simulink model "external_state_machine"  (R2021a)
settings: Solver=FixedStepDiscrete  StartTime=0.0  StopTime=2000*t_ADC  RelTol=1e-3
values from neighbouring files (symbols this model uses):
  A = 0.1    [uz_mpc_6ph_init.m]    (also in uz_mpc_6ph_state_machine_init.m)
  IB = sqrt(2)*IR    [uz_mpc_6ph_init.m]    (also in uz_mpc_6ph_state_machine_init.m)
  id_ref = 0.0    (= 0)    [uz_mpc_6ph_init.m]    (also in uz_mpc_6ph_state_machine_init.m)
  iq_ref = 15.0    (= 15)    [uz_mpc_6ph_init.m]    (also in uz_mpc_6ph_state_machine_init.m = 10)
  ix_ref = 0.0    (= 0)    [uz_mpc_6ph_init.m]    (also in uz_mpc_6ph_state_machine_init.m)
  iy_ref = 0.0    (= 0)    [uz_mpc_6ph_init.m]    (also in uz_mpc_6ph_state_machine_init.m)
  lambda_d = 1.0    (= 1)    [uz_mpc_6ph_init.m]    (also in uz_mpc_6ph_state_machine_init.m)
  lambda_q = 1.0    (= 1)    [uz_mpc_6ph_init.m]    (also in uz_mpc_6ph_state_machine_init.m)
  lambda_u = 0.0    (= 0)    [uz_mpc_6ph_init.m]    (also in uz_mpc_6ph_state_machine_init.m)
  lambda_x = 1.0    (= 1)    [uz_mpc_6ph_init.m]    (also in uz_mpc_6ph_state_machine_init.m)
  lambda_y = 1.0    (= 1)    [uz_mpc_6ph_init.m]    (also in uz_mpc_6ph_state_machine_init.m)
  Ld_over_LB = Ld/LB    [uz_mpc_6ph_init.m]    (also in uz_mpc_6ph_state_machine_init.m)
  Lq_over_LB = Lq/LB    [uz_mpc_6ph_init.m]    (also in uz_mpc_6ph_state_machine_init.m)
  n_rpm = 2200.0    (= 2200)    [uz_mpc_6ph_init.m]    (also in uz_mpc_6ph_state_machine_init.m = 100)
  omega_m = n_rpm*pi/30    (= 230.383461263)    [uz_mpc_6ph_init.m]    (also in uz_mpc_6ph_state_machine_init.m = 10.471975512)
  omegaB = nR*2*pi()/60*p    [uz_mpc_6ph_init.m]    (also in uz_mpc_6ph_state_machine_init.m)
  p = 5    [uz_mpc_6ph_init.m]    (also in uz_mpc_6ph_state_machine_init.m)
  psi_pm_over_psiB = psi_pm/psiB    [uz_mpc_6ph_init.m]    (also in uz_mpc_6ph_state_machine_init.m)
  Rs_over_ZB = Rs/ZB    [uz_mpc_6ph_init.m]    (also in uz_mpc_6ph_state_machine_init.m)
  t_ADC = 1/f_ADC    (= 1e-05)    [uz_mpc_6ph_init.m]    (also in uz_mpc_6ph_state_machine_init.m)
  t_clock = 1/f_clock    (= 1e-08)    [uz_mpc_6ph_init.m]    (also in uz_mpc_6ph_state_machine_init.m)
  Ts_times_ZB_over_Ld = Ts*ZB/Ld    [uz_mpc_6ph_init.m]    (also in uz_mpc_6ph_state_machine_init.m)
  Ts_times_ZB_over_Lq = Ts*ZB/Lq    [uz_mpc_6ph_init.m]    (also in uz_mpc_6ph_state_machine_init.m)
  Ts_times_ZB_over_Lx = Ts*ZB/Lx    [uz_mpc_6ph_init.m]    (also in uz_mpc_6ph_state_machine_init.m)
  Ts_times_ZB_over_Ly = Ts*ZB/Ly    [uz_mpc_6ph_init.m]    (also in uz_mpc_6ph_state_machine_init.m)
  v_dc = 565.0    (= 565)    [uz_mpc_6ph_init.m]    (also in uz_mpc_6ph_state_machine_init.m = 50)
  VB = sqrt(2/3)*VR    [uz_mpc_6ph_init.m]    (also in uz_mpc_6ph_state_machine_init.m)
libraries: nesl_utility x38, fl_lib x30, simulink x19, ee_lib x14, hdlsllib x4, spsAlphaBetaZerotodq0Lib x1
(part 2 of 4)

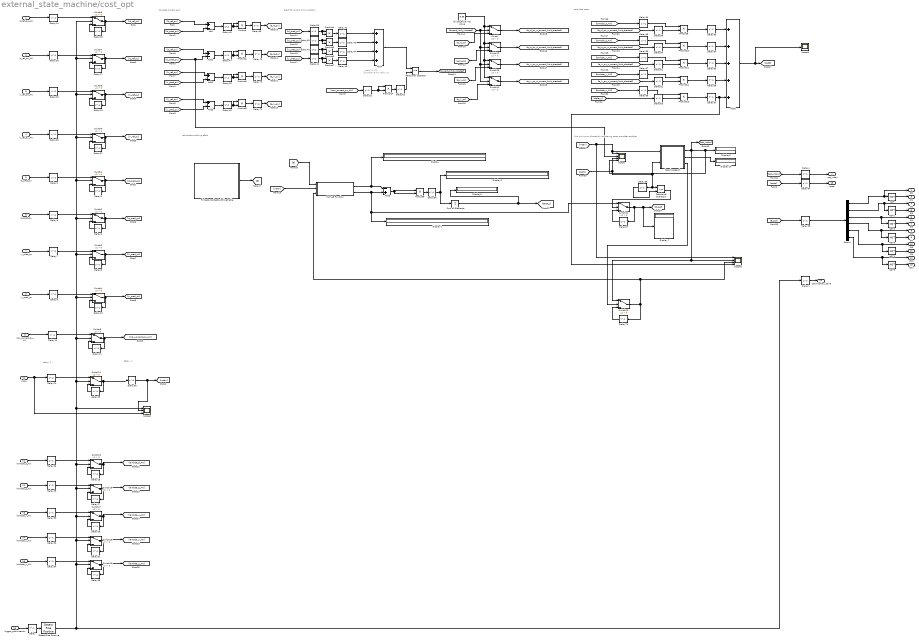
== system external_state_machine/cost_opt ==
  note: delay 4 !
  note: delay 2 !
  note: i_max^2 <= id^2+iq^2+ix^2+iy^2
  note: find minimum of costs by comparing costs one after another
  note: calculate costs
  note: calculate switching effort
  note: check for current limit violation
  note: squared current error
  id_ref_pu_AXI : Inport
  iq_ref_pu_AXI : Inport  Port=2
  ix_ref_pu_AXI : Inport  Port=3
  iy_ref_pu_AXI : Inport  Port=4
  id_pred_pu : Inport  Port=5
  iq_pred_pu : Inport  Port=6
  ix_pred_pu : Inport  Port=7
  iy_pred_pu : Inport  Port=8
  max_current_pu_AXI : Inport  Port=9
  index : Inport  Port=10
  lambda_d_AXI : Inport  Port=11
  lambda_q_AXI : Inport  Port=12
  lambda_x_AXI : Inport  Port=13
  lambda_y_AXI : Inport  Port=14
  lambda_u_AXI : Inport  Port=15
  trigger_optimization : Inport  Port=16
  Add{,1..3} (4 alike) : Sum  Inputs=+-
  Add4 : Sum  Inputs=++++  AccumDataTypeStr=fixdt_type_squared_current_error
  Add5 : Sum  Inputs=-+
  Add6 : Sum  Inputs=+++++  AccumDataTypeStr=fixdt_type_delta_u_costs
  Delay{,1..12,14..21,25..34,36,38..49,51..72,94} (67 alike) : Delay  DelayLength=1
  Delay23 : Delay  DelayLength=1  InitialCondition=1
  Delay24 : Delay  InitialCondition=1
  Delay35 : Delay  DelayLength=1  InitialCondition=4.99
  Delay37 : Delay  DelayLength=1  InitialCondition=0
  Delay50 : Delay  DelayLength=4  InitialCondition=1
  Delay73 : Delay  DelayLength=1  InitialCondition=1
  Demux : Demux  Outputs=6
  Detect Rise Positive : simulink/Logic and Bit Operations/Detect Rise Positive  vinit=0  OutDataTypeStr=boolean
  Display{,1..3,6..7,10} (7 alike) : Display
  FiniteControlSetSwitchingTable : MATLAB Function  TreatAsAtomicUnit=on
  MATLAB Function : MATLAB Function  TreatAsAtomicUnit=on
  NOT{,1..5} (6 alike) : Logic  Operator=NOT  IconShape=distinctive  AllPortsSameDT=off  OutDataTypeStr=boolean
  Product{,1..7,9..12,14} (13 alike) : Product  OutDataTypeStr=fixdt_type_squared_current_error
  Product13 : Product  OutDataTypeStr=fixdt_type_delta_u_costs
  Product8 : Product  OutDataTypeStr=uint16
  Relational Operator : RelationalOperator  OutDataTypeStr=boolean  RndMeth=Simplest
  Relational Operator1 : RelationalOperator  Operator=<=  OutDataTypeStr=boolean  RndMeth=Simplest
  Scope : Scope  NumInputPorts=4
  Scope1 : Scope  NumInputPorts=4
  Scope2 : Scope  NumInputPorts=3
  Scope3 : Scope
  Sum of Elements : Sum  Inputs=+  AccumDataTypeStr=uint16
  Switch{,1..9,11..21} (21 alike) : Switch  Criteria=u2 > Threshold
  iterativesearch : MATLAB Function  TreatAsAtomicUnit=on
  sfix18_En15 max value : Constant  Value=3.99  OutDataTypeStr=fixdt(1,18,15)  SampleTime=-1
  opt_index : Outport  VectorParamsAs1DForOutWhenUnconnected=off
  G0 : Outport  Port=2  VectorParamsAs1DForOutWhenUnconnected=off
  G1 : Outport  Port=3  VectorParamsAs1DForOutWhenUnconnected=off
  G2 : Outport  Port=4  VectorParamsAs1DForOutWhenUnconnected=off
  G3 : Outport  Port=5  VectorParamsAs1DForOutWhenUnconnected=off
  G4 : Outport  Port=6  VectorParamsAs1DForOutWhenUnconnected=off
  G5 : Outport  Port=7  VectorParamsAs1DForOutWhenUnconnected=off
  G6 : Outport  Port=8  VectorParamsAs1DForOutWhenUnconnected=off
  G7 : Outport  Port=9  VectorParamsAs1DForOutWhenUnconnected=off
  G8 : Outport  Port=10  VectorParamsAs1DForOutWhenUnconnected=off
  G9 : Outport  Port=11  VectorParamsAs1DForOutWhenUnconnected=off
  G10 : Outport  Port=12  VectorParamsAs1DForOutWhenUnconnected=off
  G11 : Outport  Port=13  VectorParamsAs1DForOutWhenUnconnected=off
  optimization_done : Outport  Port=14  VectorParamsAs1DForOutWhenUnconnected=off
  costs : Outport  Port=15  VectorParamsAs1DForOutWhenUnconnected=off
  wires:
  trigger_optimization/1 -> Delay/1
  Delay/1 -> Detect Rise Positive/1
  Delay1/1 -> optimization_done/1
  Delay4/1 -> opt_index/1
  Switch9/1 -> [iy_ref_pu], Delay21/1
  Delay17/1 -> Switch7/3
  id_ref_pu_AXI/1 -> Delay14/1
  Delay18/1 -> Switch8/1
  Switch8/1 -> [ix_ref_pu], Delay19/1
  Delay21/1 -> Switch9/3
  Switch7/1 -> [iq_ref_pu], Delay17/1
  iy_ref_pu_AXI/1 -> Delay20/1
  iq_ref_pu_AXI/1 -> Delay16/1
  Delay16/1 -> Switch7/1
  Delay19/1 -> Switch8/3
  Delay20/1 -> Switch9/1
  Delay15/1 -> Switch6/3
  Switch6/1 -> [id_ref_pu], Delay15/1
  ix_ref_pu_AXI/1 -> Delay18/1
  Delay14/1 -> Switch6/1
  Switch1/1 -> [id_pred_pu], Delay3/1
  ix_pred_pu/1 -> Delay7/1
  Delay9/1 -> Switch4/1
  Delay2/1 -> Switch1/1
  Delay8/1 -> Switch3/3
  Delay5/1 -> Switch2/1
  iy_pred_pu/1 -> Delay9/1
  iq_pred_pu/1 -> Delay5/1
  Switch3/1 -> Delay8/1, [ix_pred_pu]
  Delay10/1 -> Switch4/3
  Switch2/1 -> [iq_pred_pu], Delay6/1
  Delay7/1 -> Switch3/1
  Switch4/1 -> [iy_pred_pu], Delay10/1
  Delay6/1 -> Switch2/3
  Delay3/1 -> Switch1/3
  id_pred_pu/1 -> Delay2/1
  max_current_pu_AXI/1 -> Delay12/1
  Delay12/1 -> Switch5/1
  Delay11/1 -> Switch5/3
  Switch5/1 -> [max_current_pu_AXI], Delay11/1
  FiniteControlSetSwitchingTable/1(G) -> [G]
  Delay24/1 -> Switch11/1
  index/1 -> Scope2/3, Delay24/1
  Delay23/1 -> Switch11/3
  Switch11/1 -> Delay23/1, Delay50/1
  [e_id_pu] -> Switch/3
  [current_limit_violated] -> Switch13/2, Switch14/2, Switch12/2, Switch/2
  [e_iq_pu] -> Switch12/3
  [e_ix_pu] -> Switch13/3
  sfix18_En15 max value/1 -> Switch/1, Switch14/1, Switch13/1, Switch12/1
  [e_iy_pu] -> Switch14/3
  [G] -> MATLAB Function/1(in)
  Delay26/1 -> Switch15/1
  Delay25/1 -> Switch15/3
  Switch15/1 -> [lambda_d_AXI], Delay25/1
  lambda_d_AXI/1 -> Delay26/1
  lambda_q_AXI/1 -> Delay28/1
  Delay28/1 -> Switch16/1
  Switch16/1 -> [lambda_q_AXI], Delay27/1
  Delay27/1 -> Switch16/3
  lambda_y_AXI/1 -> Delay32/1
  Switch18/1 -> [lambda_y_AXI], Delay31/1
  Delay31/1 -> Switch18/3
  Delay32/1 -> Switch18/1
  lambda_x_AXI/1 -> Delay30/1
  Delay30/1 -> Switch17/1
  Switch17/1 -> [lambda_x_AXI], Delay29/1
  Delay29/1 -> Switch17/3
  Delay33/1 -> Switch19/3
  Switch19/1 -> [lambda_u_AXI], Delay33/1
  lambda_u_AXI/1 -> Delay34/1
  Delay34/1 -> Switch19/1
  [opt_index] -> Delay4/1
  Delay38/1 -> Demux/1
  Add4/1 -> Relational Operator/1
  NOT/1 -> G1/1
  Demux/1 -> G0/1, NOT/1
  NOT5/1 -> G11/1
  NOT4/1 -> G9/1
  NOT3/1 -> G7/1
  NOT2/1 -> G5/1
  NOT1/1 -> G3/1
  Demux/2 -> NOT1/1, G2/1
  Demux/3 -> NOT2/1, G4/1
  Demux/4 -> NOT3/1, G6/1
  Demux/5 -> NOT4/1, G8/1
  Demux/6 -> NOT5/1, G10/1
  Product8/1 -> Delay58/1
  Add5/1 -> Product8/1, Product8/2
  MATLAB Function/1(G_next) -> Display/1, Add5/1
  Product9/1 -> Delay53/1
  Product10/1 -> Delay54/1
  Product11/1 -> Delay55/1
  Product12/1 -> Delay56/1
  Product13/1 -> Delay57/1
  Add6/1 -> Scope3/1, [costs]
  [lambda_d_AXI] -> Delay64/1
  [lambda_q_AXI] -> Delay65/1
  [lambda_x_AXI] -> Delay66/1
  [lambda_y_AXI] -> Delay67/1
  [lambda_u_AXI] -> Delay68/1
  [delta_u] -> Delay63/1
  [e_id_pu_w_current_limit_checked] -> Delay59/1
  [e_iy_pu_w_current_limit_checked] -> Delay62/1
  [e_ix_pu_w_current_limit_checked] -> Delay61/1
  [e_iq_pu_w_current_limit_checked] -> Delay60/1
  [id_ref_pu] -> Add/1
  [id_pred_pu] -> Add/2
  [iq_pred_pu] -> Scope/2, Add1/2
  [iq_ref_pu] -> Add1/1
  [ix_ref_pu] -> Add2/1
  [ix_pred_pu] -> Add2/2
  [iy_ref_pu] -> Add3/1
  [iy_pred_pu] -> Add3/2
  Add3/1 -> Delay49/1
  Add1/1 -> Delay47/1
  Add2/1 -> Delay48/1
  Add/1 -> Delay46/1
  Product3/1 -> Delay72/1
  Product2/1 -> Delay71/1
  Product1/1 -> Delay70/1
  Product/1 -> Delay69/1
  Product4/1 -> Delay42/1
  Product5/1 -> Delay43/1
  Product6/1 -> Delay44/1
  Product7/1 -> Delay45/1
  [id_pred_pu] -> Delay36/1
  [iq_pred_pu] -> Delay39/1
  [ix_pred_pu] -> Delay40/1
  [iy_pred_pu] -> Delay41/1
  Relational Operator/1 -> [current_limit_violated]
  Switch14/1 -> [e_iy_pu_w_current_limit_checked]
  Switch13/1 -> [e_ix_pu_w_current_limit_checked]
  Switch12/1 -> [e_iq_pu_w_current_limit_checked]
  Switch/1 -> [e_id_pu_w_current_limit_checked]
  [max_current_pu_AXI] -> Delay51/1
  Product14/1 -> Delay52/1
  [costs] -> Delay94/1
  Delay94/1 -> costs/1
  Delay37/1 -> Switch21/3
  Switch21/1 -> Display7/1, [G_opt], Delay37/1
  Detect Rise Positive/1 -> Scope2/1, Switch4/2, Switch3/2, Switch2/2, Switch1/2, Switch6/2, Switch7/2, Switch8/2, Switch9/2, Switch5/2, Switch11/2, Switch15/2, Switch16/2, Switch17/2, Switch18/2, Switch19/2, Delay1/1
  [costs] -> Scope/3, Delay35/1, Relational Operator1/1, iterativesearch/2(cost)
  [index] -> Scope1/1, iterativesearch/1(index), Scope/1  "idx"
  Delay35/1 -> Relational Operator1/2
  Relational Operator1/1 -> Switch21/2
  [G_opt] -> Delay38/1
  Delay36/1 -> Product4/2, Product4/1
  Delay39/1 -> Product5/2, Product5/1
  Delay40/1 -> Product6/2, Product6/1
  Delay41/1 -> Product7/2, Product7/1
  Delay44/1 -> Add4/3
  Delay42/1 -> Add4/1
  Delay45/1 -> Add4/4
  Delay43/1 -> Add4/2
  Delay46/1 -> Product/1, Product/2
  Delay47/1 -> Product1/1, Product1/2
  Delay48/1 -> Product2/1, Product2/2
  Delay49/1 -> Product3/1, Product3/2
  Delay50/1 -> Scope2/2, [index]
  Delay51/1 -> Product14/1, Product14/2
  Delay52/1 -> Relational Operator/2
  Delay53/1 -> Add6/1
  Delay54/1 -> Add6/2
  Delay55/1 -> Add6/3
  Delay56/1 -> Add6/4
  Delay57/1 -> Add6/5, Scope1/4  "dU"
  Delay58/1 -> Sum of Elements/1, Display2/1
  Delay59/1 -> Product9/2
  Delay60/1 -> Product10/2
  Delay61/1 -> Product11/2
  Delay62/1 -> Product12/2
  Delay63/1 -> Product13/2
  Delay64/1 -> Product9/1
  Delay65/1 -> Product10/1
  Delay66/1 -> Product11/1
  Delay67/1 -> Product12/1
  Delay68/1 -> Product13/1
  Delay69/1 -> [e_id_pu]
  Delay70/1 -> [e_iq_pu]
  Delay71/1 -> [e_ix_pu]
  Delay72/1 -> [e_iy_pu]
  Sum of Elements/1 -> [delta_u], Display3/1
  Switch20/1 -> Delay73/1, MATLAB Function/3(last_optim_index), Scope1/3  "last_opt_idx"
  MATLAB Function/2(G_prev) -> Display1/1, Switch21/1, Add5/2
  Delay73/1 -> Switch20/3
  iterativesearch/1(opt_idx) -> Scope1/2, Switch20/1, Scope/4, Display6/1, [opt_index]  "opt_idx"
  iterativesearch/3(opt_done) -> Switch20/2
  iterativesearch/2(min_costs) -> Display10/1
  [index] -> MATLAB Function/2(index)

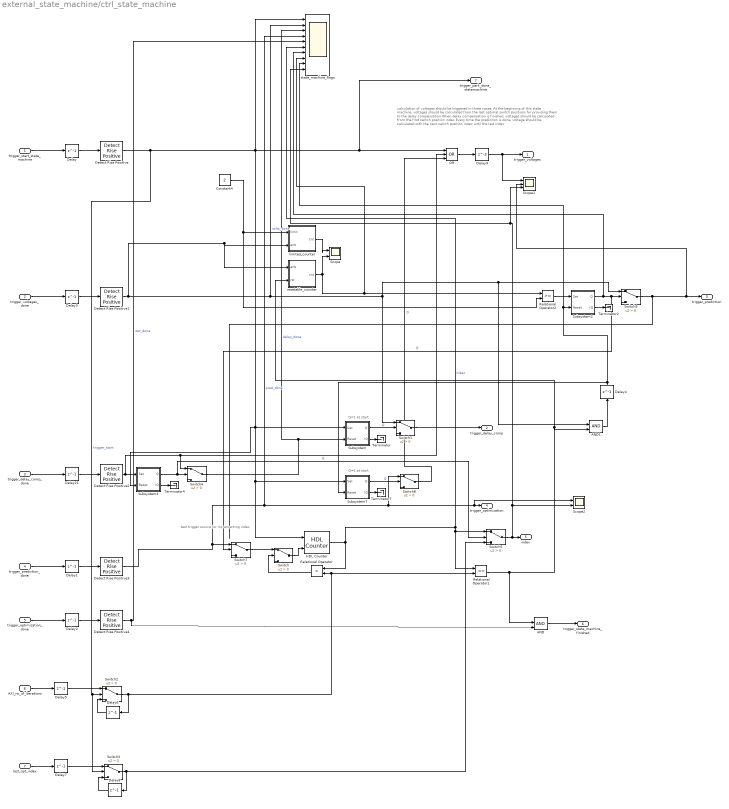
== system external_state_machine/ctrl_state_machine ==
  note: test trigger source for incrementing index
  note: calculation of voltages should be triggered in three cases:
      |
      | At the beginning of this state machine, voltages should be calculated from the last optimal switch positions for providing them to the delay compensation
      | When delay compensation is finished, voltages should be calculated from the first switch position index
      | Every time the prediciton is done, voltage should be calculated with the next switch position index until the last index
  note: Q=1 at start
  note: Q=1 at start
  trigger_start_state_machine : Inport
  trigger_voltages_done : Inport  Port=2
  trigger_delay_comp_done : Inport  Port=3
  trigger_prediction_done : Inport  Port=4
  trigger_optimization_done : Inport  Port=5
  AXI_no_of_iterations : Inport  Port=6  OutDataTypeStr=uint32
  last_opt_index : Inport  Port=7  OutDataTypeStr=uint32
  AND : Logic  IconShape=distinctive  AllPortsSameDT=off  OutDataTypeStr=boolean
  AND1 : Logic  IconShape=distinctive  AllPortsSameDT=off  OutDataTypeStr=boolean
  Constant4 : Constant  Value=2  OutDataTypeStr=uint8  SampleTime=-1
  Delay{,1..8,21} (10 alike) : Delay  DelayLength=1
  Delay9 : Delay  DelayLength=3
  Detect Rise Positive{,1..4} (5 alike) : simulink/Logic and Bit Operations/Detect Rise Positive  vinit=0  OutDataTypeStr=boolean
  HDL Counter : hdlsllib/Sources/HDL Counter  CountType=Free running  CountInit=1  CountStep=1  CountMax=25  CountFromType=Initial value  CountFrom=1  CountResetPort=on  CountLoadPort=off  CountEnbPort=on  CountDirPort=off  CountHitOutputPort=off  CountDataType=Unsigned  CountWordLen=32  CountFracLen=0  CountSampTime=1
  OR : Logic  Operator=OR  Inputs=3  IconShape=distinctive  AllPortsSameDT=off  OutDataTypeStr=boolean
  Relational Operator : RelationalOperator  Operator=<  OutDataTypeStr=boolean  RndMeth=Simplest
  Relational Operator1 : RelationalOperator  Operator===  OutDataTypeStr=boolean  RndMeth=Simplest
  Relational Operator2 : RelationalOperator  OutDataTypeStr=boolean  RndMeth=Simplest
  Scope : Scope  NumInputPorts=2
  Scope1 : Scope  NumInputPorts=3
  Scope2 : Scope  NumInputPorts=2
  Subsystem : Subsystem
  Subsystem2 : Subsystem
  Subsystem4 : Subsystem
  Subsystem7 : Subsystem
  Switch{,1..5,7..9} (9 alike) : Switch  Criteria=u2 > Threshold
  Terminator{,2,4,7} (4 alike) : Terminator
  limited_counter : Subsystem
  resetable_counter : Subsystem
  state_machine_flags : Scope  NumInputPorts=10
  trigger_voltages : Outport  VectorParamsAs1DForOutWhenUnconnected=off
  trigger_delay_comp : Outport  Port=2  VectorParamsAs1DForOutWhenUnconnected=off
  trigger_prediction : Outport  Port=3  VectorParamsAs1DForOutWhenUnconnected=off
  trigger_optimization : Outport  Port=4  VectorParamsAs1DForOutWhenUnconnected=off
  index : Outport  Port=5  VectorParamsAs1DForOutWhenUnconnected=off
  trigger_state_machine_finished : Outport  Port=6  VectorParamsAs1DForOutWhenUnconnected=off
  trigger_park_done_statemachine : Outport  Port=7  VectorParamsAs1DForOutWhenUnconnected=off
  wires:
  Switch2/1 -> Delay6/1, Relational Operator/2, Relational Operator1/2
  Relational Operator/1 -> Switch/2
  Detect Rise Positive/1 -> Switch3/2, Switch2/2, state_machine_flags/1, HDL Counter/1, Subsystem7/1(Set), Subsystem/1(Set), Subsystem4/2(Reset), trigger_park_done_statemachine/1, OR/1  "trigger_start"
  Subsystem/1(Q) -> Switch1/2  "Q"
  Subsystem/2(!Q) -> Terminator/1
  Switch1/1 -> trigger_delay_comp/1
  trigger_voltages_done/1 -> Delay3/1
  trigger_delay_comp_done/1 -> Delay21/1
  Delay21/1 -> Detect Rise Positive2/1
  Delay/1 -> Detect Rise Positive/1
  trigger_start_state_machine/1 -> Delay/1
  Delay2/1 -> Detect Rise Positive4/1
  trigger_optimization_done/1 -> Delay2/1
  Delay1/1 -> Detect Rise Positive3/1
  trigger_prediction_done/1 -> Delay1/1
  Subsystem4/1(Q) -> Switch5/2, Switch4/2  "Q"
  Subsystem4/2(!Q) -> Terminator4/1
  Detect Rise Positive2/1 -> OR/2, Switch4/1, Subsystem4/1(Set)
  Switch4/1 -> state_machine_flags/3, Subsystem/2(Reset)  "delay_done"
  Detect Rise Positive1/1 -> resetable_counter/1(enb), limited_counter/2(enb), state_machine_flags/2, AND1/1, Switch9/1, Switch1/1  "volts_done"
  Delay3/1 -> Detect Rise Positive1/1
  Subsystem2/2(!Q) -> Terminator2/1
  Subsystem2/1(Q) -> state_machine_flags/7, Switch7/2, Switch9/2  "Q"
  Constant4/1 -> Relational Operator2/2, limited_counter/1(limit)
  Relational Operator2/1 -> Subsystem2/1(Set)
  limited_counter/1(cnt) -> Scope/1
  Detect Rise Positive3/1 -> Switch7/1, state_machine_flags/4, Switch8/1, Scope2/1, trigger_optimization/1  "pred_done"
  Switch/1 -> HDL Counter/2
  HDL Counter/1 -> Switch5/1, Relational Operator1/1, state_machine_flags/6, Relational Operator/1  "index"
  Detect Rise Positive4/1 -> state_machine_flags/5, AND/2  "opt_done"
  Switch7/1 -> Switch/1
  resetable_counter/1(cnt) -> Scope/2, state_machine_flags/8, Relational Operator2/1
  Relational Operator1/1 -> AND1/2, resetable_counter/2(rst), AND/1
  Switch9/1 -> Scope1/2, trigger_prediction/1
  AND/1 -> trigger_state_machine_finished/1
  AND1/1 -> Delay4/1
  Delay4/1 -> state_machine_flags/9, Subsystem2/2(Reset), Subsystem7/2(Reset)
  Switch8/1 -> OR/3  "Q"
  Subsystem7/2(!Q) -> Terminator7/1
  Subsystem7/1(Q) -> Switch8/2  "Q"
  AXI_no_of_iterations/1 -> Delay5/1
  Delay5/1 -> Switch2/1
  Delay6/1 -> Switch2/3
  last_opt_index/1 -> Delay7/1
  Switch3/1 -> Switch5/3, Delay8/1
  Delay7/1 -> Switch3/1
  Delay8/1 -> Switch3/3
  Switch5/1 -> Scope1/3, state_machine_flags/10, Scope2/2, index/1
  OR/1 -> Delay9/1
  Delay9/1 -> Scope1/1, trigger_voltages/1

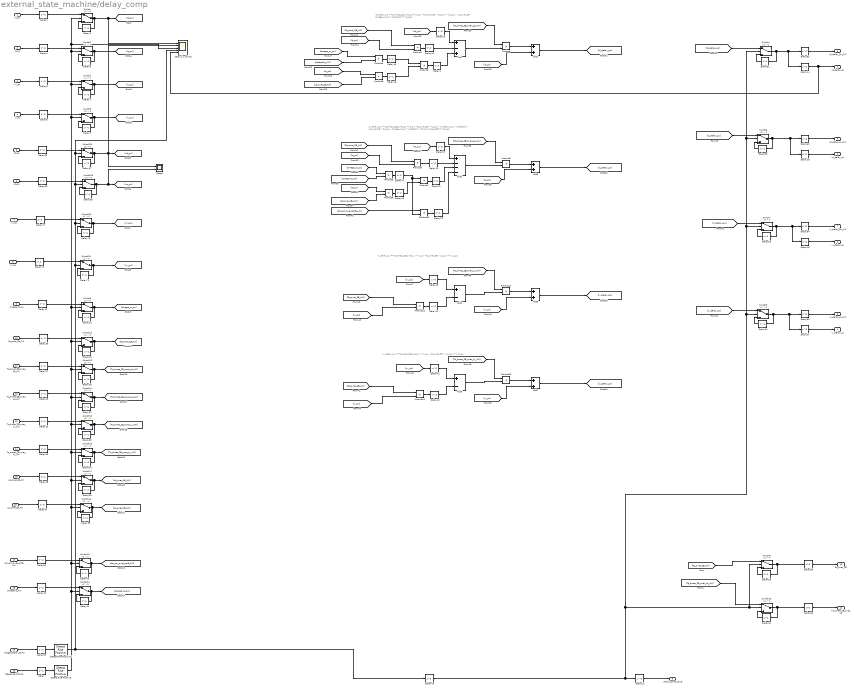
== system external_state_machine/delay_comp ==
  note: iy_delay_pu = Ts_times_ZB_over_Ly *(vy_pu - Rs_over_ZB * iy_k_pu) + iy_k_pu
  note: ix_delay_pu = Ts_times_ZB_over_Lx *(vx_pu - Rs_over_ZB* ix_k_pu) + ix_k_pu
  note: iq_delay_pu = Ts_times_ZB_over_Lq *(vq_pu - Rs_over_ZB * iq_k_pu - omega_m_pu * polepairs * Ld_over_LB * id_k_pu - omega_m_pu * polepairs * psi_pm_over_psiB) + iq_k_pu
  note: id_delay_pu = Ts_times_ZB_over_Ld *(vd_pu - Rs_over_ZB * id_k_pu + iq_k_pu * Lq_over_LB * omega_m_pu * polepairs) + id_k_pu
  id_pu : Inport  OutDataTypeStr=fixdt_type_dq_currents
  iq_pu : Inport  Port=2  OutDataTypeStr=fixdt_type_dq_currents
  ix_pu : Inport  Port=3  OutDataTypeStr=fixdt_type_xy_currents
  iy_pu : Inport  Port=4  OutDataTypeStr=fixdt_type_xy_currents
  vd_pu : Inport  Port=5  OutDataTypeStr=fixdt_type_dqxy_voltages
  vq_pu : Inport  Port=6  OutDataTypeStr=fixdt_type_dqxy_voltages
  vx_pu : Inport  Port=7  OutDataTypeStr=fixdt_type_dqxy_voltages
  vy_pu : Inport  Port=8  OutDataTypeStr=fixdt_type_dqxy_voltages
  omega_m_pu : Inport  Port=9  OutDataTypeStr=fixdt_type_speed
  Rs_over_ZB_AXI : Inport  Port=10  OutDataTypeStr=fixdt_type_constants
  Ts_times_ZB_over_Ld_AXI : Inport  Port=11  OutDataTypeStr=fixdt_type_constants
  Ts_times_ZB_over_Lq_AXI : Inport  Port=12  OutDataTypeStr=fixdt_type_constants
  Ts_times_ZB_over_Lx_AXI : Inport  Port=13  OutDataTypeStr=fixdt_type_constants
  Ts_times_ZB_over_Ly_AXI : Inport  Port=14  OutDataTypeStr=fixdt_type_constants
  Ld_over_LB_AXI : Inport  Port=15  OutDataTypeStr=fixdt_type_constants
  Lq_over_LB_AXI : Inport  Port=16  OutDataTypeStr=fixdt_type_constants
  psi_pm_over_psiB_AXI : Inport  Port=17  OutDataTypeStr=fixdt_type_constants
  polepairs_AXI : Inport  Port=18  OutDataTypeStr=fixdt_type_polepairs
  trigger_delay_comp : Inport  Port=19
  trigger_park_done : Inport  Port=20
  Add : Sum  Inputs=+-+  AccumDataTypeStr=fixdt(1,27,16)
  Add{1,3,5,7} (4 alike) : Sum  AccumDataTypeStr=fixdt(1,27,24)
  Add2 : Sum  Inputs=+---  AccumDataTypeStr=fixdt(1,27,16)
  Add4 : Sum  Inputs=+-  AccumDataTypeStr=fixdt(1,27,16)
  Add6 : Sum  Inputs=+-  AccumDataTypeStr=fixdt(1,27,16)
  Delay{,2,4,6,8,10..12,14..20,23..25,27,29,31,33,35,37,39,41..43,49..50,56,59..60,62..66,71,73} (40 alike) : Delay
  Delay{1,3,5,7,9,13,21..22,26,28,30,32,34,36,38,40,44..48,51..55,57..58,61,70,72} (31 alike) : Delay  DelayLength=1
  Detect Rise Positive : simulink/Logic and Bit Operations/Detect Rise Positive  vinit=0  OutDataTypeStr=boolean
  Detect Rise Positive1 : simulink/Logic and Bit Operations/Detect Rise Positive  vinit=0  OutDataTypeStr=boolean
  Product{,1..2,4..7,9..14} (13 alike) : Product  OutDataTypeStr=fixdt(1,18,15)
  Product3 : Product  OutDataTypeStr=fixdt(1,27,16)
  Product8 : Product  OutDataTypeStr=fixdt(1,27,16)
  Scope : Scope  NumInputPorts=2
  Switch : Switch  Criteria=u2 > Threshold  OutDataTypeStr=fixdt_type_dq_currents
  Switch1 : Switch  Criteria=u2 > Threshold  OutDataTypeStr=fixdt_type_dq_currents
  Switch{4,6..10} (6 alike) : Switch  Criteria=u2 > Threshold
  Switch{12..19} (8 alike) : Switch  Criteria=u2 > Threshold  OutDataTypeStr=fixdt_type_constants
  Switch2 : Switch  Criteria=u2 > Threshold  OutDataTypeStr=fixdt_type_xy_currents
  Switch21 : Switch  Criteria=u2 > Threshold  OutDataTypeStr=fixdt_type_polepairs
  Switch{28..31} (4 alike) : Switch  Criteria=u2 > Threshold  OutDataTypeStr=fixdt_type_dqxy_voltages
  Switch3 : Switch  Criteria=u2 > Threshold  OutDataTypeStr=fixdt_type_xy_currents
  Switch5 : Switch  Criteria=u2 > Threshold  OutDataTypeStr=fixdt_type_speed
  delay_in_values : Scope  NumInputPorts=5
  id_delay_pu : Outport
  iq_delay_pu : Outport  Port=2
  ix_delay_pu : Outport  Port=3
  iy_delay_pu : Outport  Port=4
  id_delay_pu_AXI : Outport  Port=5
  iq_delay_pu_AXI : Outport  Port=6
  ix_delay_pu_AXI : Outport  Port=7
  iy_delay_pu_AXI : Outport  Port=8
  delay_comp_done : Outport  Port=9
  Rs_over_ZB : Outport  Port=10
  Ts_times_ZB_over_Ld : Outport  Port=11
  wires:
  Add5/1 -> [ix_delay_pu]
  Switch12/1 -> [Rs_over_ZB_AXI], Delay26/1
  Add3/1 -> [iq_delay_pu]
  Add1/1 -> [id_delay_pu]
  Add7/1 -> [iy_delay_pu]
  Delay5/1 -> Switch1/3
  Delay25/1 -> Switch12/1
  Delay59/1 -> Switch28/1
  Delay33/1 -> Switch16/1
  vx_pu/1 -> Delay71/1
  vd_pu/1 -> Delay59/1
  Switch15/1 -> [Ts_times_ZB_over_Lx_AXI], Delay32/1
  Ld_over_LB_AXI/1 -> Delay35/1
  Delay2/1 -> Switch/1
  Switch16/1 -> Delay34/1, [Ts_times_ZB_over_Ly_AXI]
  ix_pu/1 -> Delay6/1
  Delay38/1 -> Switch18/3
  Switch17/1 -> Delay36/1, [Ld_over_LB_AXI]
  Delay9/1 -> Switch3/3
  Switch13/1 -> [Ts_times_ZB_over_Ld_AXI], Delay28/1
  Delay/1 -> Detect Rise Positive/1
  Delay34/1 -> Switch16/3
  Delay44/1 -> Switch21/3
  Delay29/1 -> Switch14/1
  Delay8/1 -> Switch3/1
  Switch29/1 -> Scope/2, [vq_pu], Delay58/1
  Switch3/1 -> [iy_pu], Delay9/1
  polepairs_AXI/1 -> Delay43/1
  Delay72/1 -> Switch31/3
  Delay43/1 -> Switch21/1
  Switch14/1 -> [Ts_times_ZB_over_Lq_AXI], Delay30/1
  Delay28/1 -> Switch13/3
  psi_pm_over_psiB_AXI/1 -> Delay39/1
  Delay58/1 -> Switch29/3
  id_pu/1 -> Delay2/1
  Switch21/1 -> [polepairs_AXI], Delay44/1
  Switch/1 -> delay_in_values/1, [id_pu], Delay3/1
  Delay35/1 -> Switch17/1
  Delay31/1 -> Switch15/1
  Switch28/1 -> Scope/1, delay_in_values/2, [vd_pu], Delay57/1
  Ts_times_ZB_over_Ly_AXI/1 -> Delay33/1
  Delay7/1 -> Switch2/3
  Delay37/1 -> Switch18/1
  Delay4/1 -> Switch1/1
  Switch2/1 -> [ix_pu], Delay7/1
  Delay12/1 -> Switch5/1
  Delay73/1 -> Switch31/1
  Switch31/1 -> Delay72/1, [vy_pu]
  omega_m_pu/1 -> Delay12/1
  Delay6/1 -> Switch2/1
  Delay27/1 -> Switch13/1
  vq_pu/1 -> Delay60/1
  Switch5/1 -> [omega_m_pu], Delay13/1
  Lq_over_LB_AXI/1 -> Delay37/1
  iq_pu/1 -> Delay4/1
  iy_pu/1 -> Delay8/1
  vy_pu/1 -> Delay73/1
  Delay70/1 -> Switch30/3
  Delay60/1 -> Switch29/1
  Switch30/1 -> Delay70/1, [vx_pu]
  Ts_times_ZB_over_Lq_AXI/1 -> Delay29/1
  Delay3/1 -> Switch/3
  Switch18/1 -> Delay38/1, [Lq_over_LB_AXI]
  Delay26/1 -> Switch12/3
  Switch19/1 -> [psi_pm_over_psiB_AXI], Delay40/1
  Ts_times_ZB_over_Lx_AXI/1 -> Delay31/1
  Delay71/1 -> Switch30/1
  Switch1/1 -> [iq_pu], Delay5/1
  Ts_times_ZB_over_Ld_AXI/1 -> Delay27/1
  Delay57/1 -> Switch28/3
  Rs_over_ZB_AXI/1 -> Delay25/1
  Delay39/1 -> Switch19/1
  trigger_park_done/1 -> Delay/1
  Delay40/1 -> Switch19/3
  Delay13/1 -> Switch5/3
  Delay32/1 -> Switch15/3
  Delay36/1 -> Switch17/3
  Delay30/1 -> Switch14/3
  Delay11/1 -> delay_comp_done/1
  Switch8/1 -> Delay54/1, Delay17/1, Delay65/1
  Switch4/1 -> Delay51/1, Delay14/1, Delay62/1
  Delay63/1 -> iq_delay_pu_AXI/1
  Delay65/1 -> iy_delay_pu_AXI/1
  Delay64/1 -> ix_delay_pu_AXI/1
  Switch7/1 -> Delay53/1, Delay16/1, Delay64/1
  Delay62/1 -> id_delay_pu_AXI/1
  Delay15/1 -> iq_delay_pu/1
  Delay14/1 -> delay_in_values/5, id_delay_pu/1
  Delay16/1 -> ix_delay_pu/1
  Delay17/1 -> iy_delay_pu/1
  Add/1 -> Product/2
  [Ts_times_ZB_over_Ld_AXI] -> Product/1  "Ts_times_ZB_over_Ld"
  Product/1 -> Add1/1
  [id_pu] -> Add1/2  "id_k_pu"
  [Rs_over_ZB_AXI] -> Product1/1  "Rs_over_ZB"
  [id_pu] -> Product1/2  "id_k_pu"
  [iq_pu] -> Product3/1  "iq_k_pu"
  [Lq_over_LB_AXI] -> Product3/2  "Lq_over_LB"
  [omega_m_pu] -> Product4/1  "omega_m_pu"
  [polepairs_AXI] -> Product4/2  "polepairs"
  [Ts_times_ZB_over_Lq_AXI] -> Product5/1  "Ts_times_ZB_over_Lq"
  [iq_pu] -> Product6/2  "iq_k_pu"
  [Rs_over_ZB_AXI] -> Product6/1  "Rs_over_ZB"
  Add2/1 -> Product5/2
  [omega_m_pu] -> Product9/1  "omega_m_pu"
  [iq_pu] -> Add3/2  "iq_k_pu"
  [id_pu] -> Product8/1  "id_k_pu"
  [Ld_over_LB_AXI] -> Product8/2  "Ld_over_LB"
  [polepairs_AXI] -> Product9/2  "polepairs"
  Product5/1 -> Add3/1
  [psi_pm_over_psiB_AXI] -> Product10/1
  [Ts_times_ZB_over_Lx_AXI] -> Product11/1  "Ts_times_ZB_over_Lx"
  [ix_pu] -> Product12/2  "ix_k_pu"
  [Rs_over_ZB_AXI] -> Product12/1  "Rs_over_ZB"
  Add4/1 -> Product11/2
  [ix_pu] -> Add5/2  "ix_k_pu"
  Product11/1 -> Add5/1
  [Rs_over_ZB_AXI] -> Product14/1  "Rs_over_ZB"
  Add6/1 -> Product13/2
  [iy_pu] -> Add7/2  "iy_k_pu"
  [iy_pu] -> Product14/2  "iy_k_pu"
  [Ts_times_ZB_over_Ly_AXI] -> Product13/1  "Ts_times_ZB_over_Ly"
  Product13/1 -> Add7/1
  Product2/1 -> Delay1/1
  Product1/1 -> Delay10/1
  Delay10/1 -> Add/2
  Delay1/1 -> Add/3
  [vd_pu] -> Delay18/1  "vd_pu"
  Delay18/1 -> Add/1
  [vq_pu] -> Delay19/1  "vq_pu"
  Product7/1 -> Delay21/1
  Product10/1 -> Delay22/1
  Delay22/1 -> Add2/4
  Delay21/1 -> Add2/3
  Delay20/1 -> Add2/2
  Delay19/1 -> Add2/1
  Product6/1 -> Delay20/1
  [vx_pu] -> Delay23/1  "vx_pu"
  Delay23/1 -> Add4/1
  Product12/1 -> Delay24/1
  Delay24/1 -> Add4/2
  [vy_pu] -> Delay41/1  "vy_pu"
  Product14/1 -> Delay42/1
  Delay42/1 -> Add6/2
  Delay41/1 -> Add6/1
  Product4/1 -> Delay45/1
  Product3/1 -> Delay46/1
  Delay46/1 -> Product2/2
  Delay45/1 -> Product2/1
  Product9/1 -> Delay47/1
  Delay47/1 -> Product10/2, Product7/1
  Product8/1 -> Delay48/1
  Delay48/1 -> Product7/2
  trigger_delay_comp/1 -> Delay50/1
  Delay50/1 -> Detect Rise Positive1/1
  Detect Rise Positive/1 -> Switch21/2, Switch19/2, Switch18/2, Switch17/2, Switch16/2, Switch15/2, Switch14/2, Switch13/2, Switch12/2, Switch5/2, Switch3/2, Switch2/2, Switch1/2, Switch/2, delay_in_values/3
  Detect Rise Positive1/1 -> Delay49/1, delay_in_values/4, Switch28/2, Switch29/2, Switch30/2, Switch31/2  "delay_comp done"
  [id_delay_pu] -> Switch4/1
  Delay51/1 -> Switch4/3
  [iq_delay_pu] -> Switch6/1
  Switch6/1 -> Delay52/1, Delay15/1, Delay63/1
  Delay52/1 -> Switch6/3
  [ix_delay_pu] -> Switch7/1
  Delay53/1 -> Switch7/3
  Delay54/1 -> Switch8/3
  [iy_delay_pu] -> Switch8/1
  Switch9/1 -> Delay55/1, Delay56/1
  Delay55/1 -> Switch9/3
  [Rs_over_ZB_AXI] -> Switch9/1
  Delay49/1 -> Switch9/2, Switch10/2, Switch8/2, Switch7/2, Switch6/2, Switch4/2, Delay11/1
  Delay56/1 -> Rs_over_ZB/1
  Switch10/1 -> Delay61/1, Delay66/1
  Delay61/1 -> Switch10/3
  [Ts_times_ZB_over_Ld_AXI] -> Switch10/1
  Delay66/1 -> Ts_times_ZB_over_Ld/1

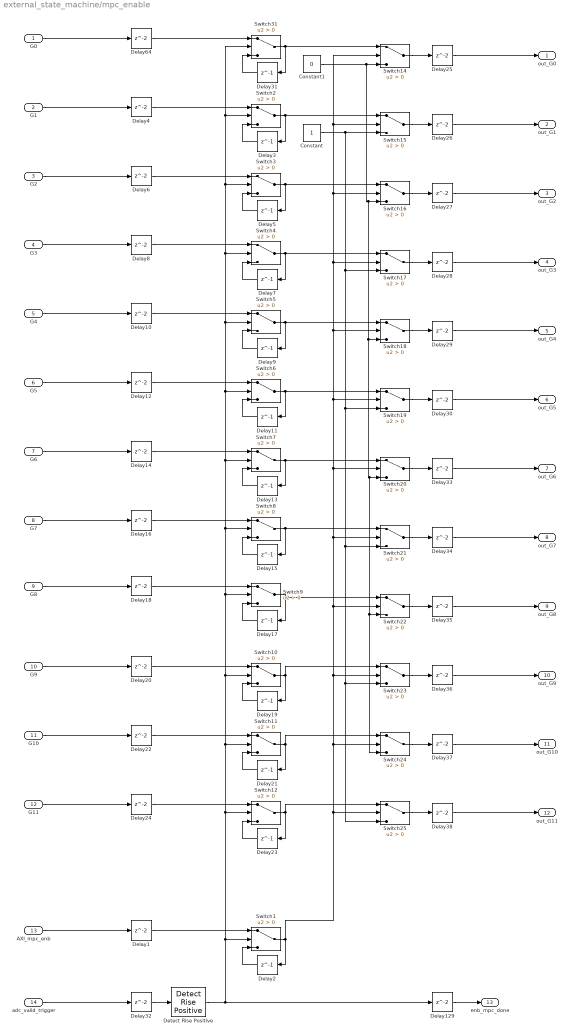
== system external_state_machine/mpc_enable ==
  G0 : Inport
  G1 : Inport  Port=2
  G2 : Inport  Port=3
  G3 : Inport  Port=4
  G4 : Inport  Port=5
  G5 : Inport  Port=6
  G6 : Inport  Port=7
  G7 : Inport  Port=8
  G8 : Inport  Port=9
  G9 : Inport  Port=10
  G10 : Inport  Port=11
  G11 : Inport  Port=12
  AXI_mpc_enb : Inport  Port=13
  adc_valid_trigger : Inport  Port=14  OutDataTypeStr=boolean
  Constant : Constant  OutDataTypeStr=boolean
  Constant1 : Constant  Value=0  OutDataTypeStr=boolean
  Delay{1,4,6,8,10,12,14,16,18,20,22,24..30,32..38,64,129} (27 alike) : Delay
  Delay{2..3,5,7,9,11,13,15,17,19,21,23,31} (13 alike) : Delay  DelayLength=1
  Detect Rise Positive : simulink/Logic and Bit Operations/Detect Rise Positive  vinit=0  OutDataTypeStr=boolean
  Switch{1..12,14..25,31} (25 alike) : Switch  Criteria=u2 > Threshold
  out_G0 : Outport
  out_G1 : Outport  Port=2
  out_G2 : Outport  Port=3
  out_G3 : Outport  Port=4
  out_G4 : Outport  Port=5
  out_G5 : Outport  Port=6
  out_G6 : Outport  Port=7
  out_G7 : Outport  Port=8
  out_G8 : Outport  Port=9
  out_G9 : Outport  Port=10
  out_G10 : Outport  Port=11
  out_G11 : Outport  Port=12
  enb_mpc_done : Outport  Port=13  OutDataTypeStr=boolean  LockScale=on
  wires:
  adc_valid_trigger/1 -> Delay32/1
  G0/1 -> Delay64/1
  Delay129/1 -> enb_mpc_done/1
  Delay64/1 -> Switch31/1
  Delay32/1 -> Detect Rise Positive/1
  Switch31/1 -> Switch14/1, Delay31/1
  Delay31/1 -> Switch31/3
  AXI_mpc_enb/1 -> Delay1/1
  Delay1/1 -> Switch1/1
  Delay2/1 -> Switch1/3
  Delay3/1 -> Switch2/3
  Switch2/1 -> Switch15/1, Delay3/1
  Delay4/1 -> Switch2/1
  G1/1 -> Delay4/1
  Detect Rise Positive/1 -> Delay129/1, Switch31/2, Switch2/2, Switch3/2, Switch4/2, Switch5/2, Switch6/2, Switch7/2, Switch8/2, Switch9/2, Switch10/2, Switch11/2, Switch12/2, Switch1/2
  Delay5/1 -> Switch3/3
  Switch3/1 -> Switch16/1, Delay5/1
  Delay6/1 -> Switch3/1
  G2/1 -> Delay6/1
  Delay7/1 -> Switch4/3
  Switch4/1 -> Switch17/1, Delay7/1
  Delay8/1 -> Switch4/1
  G3/1 -> Delay8/1
  Delay9/1 -> Switch5/3
  Switch5/1 -> Switch18/1, Delay9/1
  Delay10/1 -> Switch5/1
  G4/1 -> Delay10/1
  Delay11/1 -> Switch6/3
  Switch6/1 -> Switch19/1, Delay11/1
  Delay12/1 -> Switch6/1
  G5/1 -> Delay12/1
  Delay13/1 -> Switch7/3
  Switch7/1 -> Switch20/1, Delay13/1
  Delay14/1 -> Switch7/1
  G6/1 -> Delay14/1
  Delay15/1 -> Switch8/3
  Switch8/1 -> Switch21/1, Delay15/1
  Delay16/1 -> Switch8/1
  G7/1 -> Delay16/1
  Delay17/1 -> Switch9/3
  Switch9/1 -> Switch22/1, Delay17/1
  Delay18/1 -> Switch9/1
  G8/1 -> Delay18/1
  Delay19/1 -> Switch10/3
  Switch10/1 -> Delay19/1, Switch23/1
  Delay20/1 -> Switch10/1
  G9/1 -> Delay20/1
  Delay21/1 -> Switch11/3
  Switch11/1 -> Switch24/1, Delay21/1
  Delay22/1 -> Switch11/1
  G10/1 -> Delay22/1
  Delay23/1 -> Switch12/3
  Switch12/1 -> Switch25/1, Delay23/1
  Delay24/1 -> Switch12/1
  G11/1 -> Delay24/1
  Switch14/1 -> Delay25/1
  Delay25/1 -> out_G0/1
  Constant1/1 -> Switch24/3, Switch22/3, Switch20/3, Switch18/3, Switch16/3, Switch14/3
  Switch15/1 -> Delay26/1
  Delay26/1 -> out_G1/1
  Switch1/1 -> Switch25/2, Switch24/2, Switch23/2, Switch22/2, Switch21/2, Switch20/2, Switch19/2, Switch18/2, Switch17/2, Switch16/2, Switch15/2, Switch14/2, Delay2/1
  Switch16/1 -> Delay27/1
  Delay28/1 -> out_G3/1
  Switch17/1 -> Delay28/1
  Delay27/1 -> out_G2/1
  Delay29/1 -> out_G4/1
  Switch19/1 -> Delay30/1
  Switch18/1 -> Delay29/1
  Delay30/1 -> out_G5/1
  Switch22/1 -> Delay35/1
  Switch20/1 -> Delay33/1
  Delay35/1 -> out_G8/1
  Switch23/1 -> Delay36/1
  Delay33/1 -> out_G6/1
  Delay36/1 -> out_G9/1
  Delay38/1 -> out_G11/1
  Switch25/1 -> Delay38/1
  Switch24/1 -> Delay37/1
  Delay34/1 -> out_G7/1
  Delay37/1 -> out_G10/1
  Switch21/1 -> Delay34/1
  Constant/1 -> Switch25/3, Switch23/3, Switch21/3, Switch19/3, Switch17/3, Switch15/3

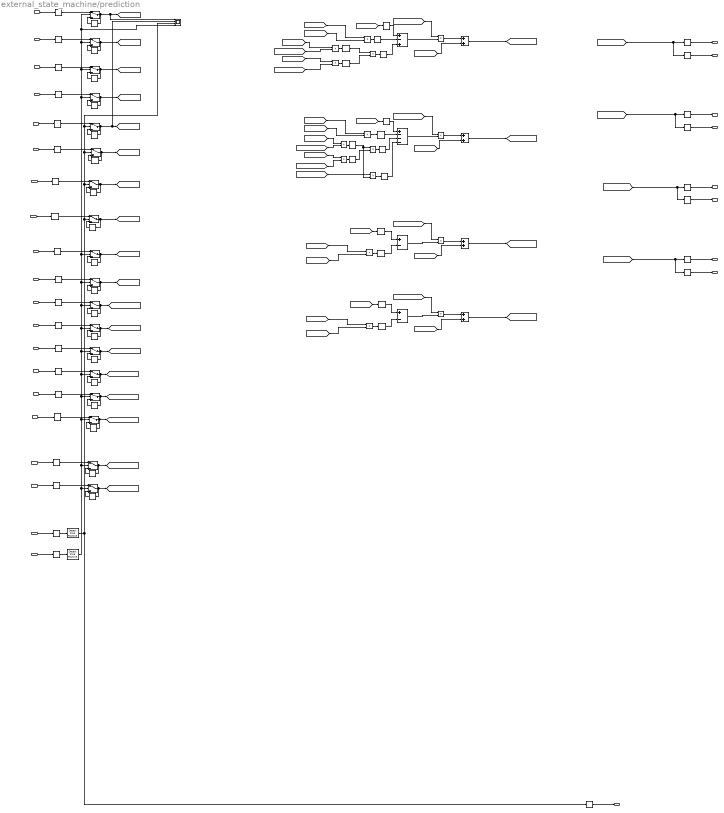
== system external_state_machine/prediction ==
  note: voltages are triggered every iteration
  note: iy_delay_pu = Ts_times_ZB_over_Ly *(vy_pu - Rs_over_ZB * iy_k_pu) + iy_k_pu
  note: ix_delay_pu = Ts_times_ZB_over_Lx *(vx_pu - Rs_over_ZB* ix_k_pu) + ix_k_pu
  note: iq_delay_pu = Ts_times_ZB_over_Lq *(vq_pu - Rs_over_ZB * iq_k_pu - omega_m_pu * polepairs * Ld_over_LB * id_k_pu - omega_m_pu * polepairs * psi_pm_over_psiB) + iq_k_pu
  note: id_delay_pu = Ts_times_ZB_over_Ld *(vd_pu - Rs_over_ZB * id_k_pu + iq_k_pu * Lq_over_LB * omega_m_pu * polepairs) + id_k_pu
  id_delay_pu : Inport  OutDataTypeStr=fixdt_type_dq_currents
  iq_delay_pu : Inport  Port=2  OutDataTypeStr=fixdt_type_dq_currents
  ix_delay_pu : Inport  Port=3  OutDataTypeStr=fixdt_type_dq_currents
  iy_delay_pu : Inport  Port=4  OutDataTypeStr=fixdt_type_dq_currents
  vd_pu : Inport  Port=5  OutDataTypeStr=fixdt_type_dqxy_voltages
  vq_pu : Inport  Port=6  OutDataTypeStr=fixdt_type_dqxy_voltages
  vx_pu : Inport  Port=7  OutDataTypeStr=fixdt_type_dqxy_voltages
  vy_pu : Inport  Port=8  OutDataTypeStr=fixdt_type_dqxy_voltages
  omega_m_pu : Inport  Port=9  OutDataTypeStr=fixdt_type_speed
  Rs_over_ZB_AXI : Inport  Port=10  OutDataTypeStr=fixdt_type_constants
  Ts_times_ZB_over_Ld_AXI : Inport  Port=11  OutDataTypeStr=fixdt_type_constants
  Ts_times_ZB_over_Lq_AXI : Inport  Port=12  OutDataTypeStr=fixdt_type_constants
  Ts_times_ZB_over_Lx_AXI : Inport  Port=13  OutDataTypeStr=fixdt_type_constants
  Ts_times_ZB_over_Ly_AXI : Inport  Port=14  OutDataTypeStr=fixdt_type_constants
  Ld_over_LB_AXI : Inport  Port=15  OutDataTypeStr=fixdt_type_constants
  Lq_over_LB_AXI : Inport  Port=16  OutDataTypeStr=fixdt_type_constants
  psi_pm_over_psiB_AXI : Inport  Port=17  OutDataTypeStr=fixdt_type_constants
  polepairs_AXI : Inport  Port=18  OutDataTypeStr=fixdt_type_polepairs
  trigger_prediction : Inport  Port=19
  trigger_delay_comp_done : Inport  Port=20
  Add : Sum  Inputs=+-+  AccumDataTypeStr=fixdt(1,27,16)
  Add{1,3,5,7} (4 alike) : Sum  AccumDataTypeStr=fixdt(1,27,24)
  Add2 : Sum  Inputs=+---  AccumDataTypeStr=fixdt(1,27,16)
  Add4 : Sum  Inputs=+-  AccumDataTypeStr=fixdt(1,27,16)
  Add6 : Sum  Inputs=+-  AccumDataTypeStr=fixdt(1,27,16)
  Delay{,2,4,6,8,11..12,14..17,25,27,29,31,33,35,37,39,43,50,59..60,62..65,71,73} (29 alike) : Delay
  Delay{1,3,5,7,9..10,13,18..24,26,28,30,32,34,36,38,40..42,44..48,57..58,70,72} (33 alike) : Delay  DelayLength=1
  Detect Rise Positive : simulink/Logic and Bit Operations/Detect Rise Positive  vinit=0  OutDataTypeStr=boolean
  Detect Rise Positive1 : simulink/Logic and Bit Operations/Detect Rise Positive  vinit=0  OutDataTypeStr=boolean
  Product{,1..2,4..7,9..14} (13 alike) : Product  OutDataTypeStr=fixdt(1,18,15)
  Product3 : Product  OutDataTypeStr=fixdt(1,27,16)
  Product8 : Product  OutDataTypeStr=fixdt(1,27,16)
  Scope : Scope  NumInputPorts=4
  Switch{,1..3} (4 alike) : Switch  Criteria=u2 > Threshold  OutDataTypeStr=fixdt_type_dq_currents
  Switch{12..19} (8 alike) : Switch  Criteria=u2 > Threshold  OutDataTypeStr=fixdt_type_constants
  Switch21 : Switch  Criteria=u2 > Threshold  OutDataTypeStr=fixdt_type_polepairs
  Switch{28..31} (4 alike) : Switch  Criteria=u2 > Threshold  OutDataTypeStr=fixdt_type_dqxy_voltages
  Switch5 : Switch  Criteria=u2 > Threshold  OutDataTypeStr=fixdt_type_speed
  id_pred_pu : Outport
  iq_pred_pu : Outport  Port=2
  ix_pred_pu : Outport  Port=3
  iy_pred_pu : Outport  Port=4
  id_pred_pu_AXI : Outport  Port=5
  iq_pred_pu_AXI : Outport  Port=6
  ix_pred_pu_AXI : Outport  Port=7
  iy_pred_pu_AXI : Outport  Port=8
  prediction_done : Outport  Port=9
  wires:
  Add5/1 -> [ix_delay_pu]
  Switch12/1 -> [Rs_over_ZB_AXI], Delay26/1
  Add3/1 -> [iq_delay_pu]
  Add1/1 -> [id_delay_pu]
  Add7/1 -> [iy_delay_pu]
  Delay5/1 -> Switch1/3
  Delay25/1 -> Switch12/1
  Delay59/1 -> Switch28/1
  Delay33/1 -> Switch16/1
  vx_pu/1 -> Delay71/1
  vd_pu/1 -> Delay59/1
  Switch15/1 -> [Ts_times_ZB_over_Lx_AXI], Delay32/1
  Ld_over_LB_AXI/1 -> Delay35/1
  Delay2/1 -> Switch/1
  Switch16/1 -> Delay34/1, [Ts_times_ZB_over_Ly_AXI]
  ix_delay_pu/1 -> Delay6/1
  Delay38/1 -> Switch18/3
  Switch17/1 -> Delay36/1, [Ld_over_LB_AXI]
  Delay9/1 -> Switch3/3
  Switch13/1 -> [Ts_times_ZB_over_Ld_AXI], Delay28/1
  Delay/1 -> Detect Rise Positive/1
  Delay34/1 -> Switch16/3
  Delay44/1 -> Switch21/3
  Delay29/1 -> Switch14/1
  Delay8/1 -> Switch3/1
  Switch29/1 -> [vq_pu], Delay58/1
  Switch3/1 -> [iy_pu], Delay9/1
  polepairs_AXI/1 -> Delay43/1
  Delay72/1 -> Switch31/3
  Delay43/1 -> Switch21/1
  Switch14/1 -> [Ts_times_ZB_over_Lq_AXI], Delay30/1
  Delay28/1 -> Switch13/3
  psi_pm_over_psiB_AXI/1 -> Delay39/1
  Delay58/1 -> Switch29/3
  id_delay_pu/1 -> Delay2/1
  Switch21/1 -> [polepairs_AXI], Delay44/1
  Switch/1 -> Scope/1, [id_pu], Delay3/1
  Delay35/1 -> Switch17/1
  Delay31/1 -> Switch15/1
  Switch28/1 -> Scope/2, [vd_pu], Delay57/1
  Ts_times_ZB_over_Ly_AXI/1 -> Delay33/1
  Delay7/1 -> Switch2/3
  Delay37/1 -> Switch18/1
  Delay4/1 -> Switch1/1
  Switch2/1 -> [ix_pu], Delay7/1
  Delay12/1 -> Switch5/1
  Delay73/1 -> Switch31/1
  Switch31/1 -> Delay72/1, [vy_pu]
  omega_m_pu/1 -> Delay12/1
  Delay6/1 -> Switch2/1
  Delay27/1 -> Switch13/1
  vq_pu/1 -> Delay60/1
  Switch5/1 -> [omega_m_pu], Delay13/1
  Lq_over_LB_AXI/1 -> Delay37/1
  iq_delay_pu/1 -> Delay4/1
  iy_delay_pu/1 -> Delay8/1
  vy_pu/1 -> Delay73/1
  Delay70/1 -> Switch30/3
  Delay60/1 -> Switch29/1
  Switch30/1 -> Delay70/1, [vx_pu]
  Ts_times_ZB_over_Lq_AXI/1 -> Delay29/1
  Delay3/1 -> Switch/3
  Switch18/1 -> Delay38/1, [Lq_over_LB_AXI]
  Delay26/1 -> Switch12/3
  Switch19/1 -> [psi_pm_over_psiB_AXI], Delay40/1
  Ts_times_ZB_over_Lx_AXI/1 -> Delay31/1
  Delay71/1 -> Switch30/1
  Switch1/1 -> [iq_pu], Delay5/1
  Ts_times_ZB_over_Ld_AXI/1 -> Delay27/1
  Delay57/1 -> Switch28/3
  Rs_over_ZB_AXI/1 -> Delay25/1
  Delay39/1 -> Switch19/1
  trigger_delay_comp_done/1 -> Delay/1
  Delay40/1 -> Switch19/3
  Delay13/1 -> Switch5/3
  Delay32/1 -> Switch15/3
  Delay36/1 -> Switch17/3
  Delay30/1 -> Switch14/3
  Delay11/1 -> prediction_done/1
  [iy_delay_pu] -> Delay17/1, Delay65/1
  [iq_delay_pu] -> Delay15/1, Delay63/1
  [id_delay_pu] -> Delay14/1, Delay62/1
  Delay63/1 -> iq_pred_pu_AXI/1
  Delay65/1 -> iy_pred_pu_AXI/1
  Delay64/1 -> ix_pred_pu_AXI/1
  [ix_delay_pu] -> Delay16/1, Delay64/1
  Delay62/1 -> id_pred_pu_AXI/1
  Delay15/1 -> iq_pred_pu/1
  Delay14/1 -> id_pred_pu/1
  Delay16/1 -> ix_pred_pu/1
  Delay17/1 -> iy_pred_pu/1
  Add/1 -> Product/2
  [Ts_times_ZB_over_Ld_AXI] -> Product/1  "Ts_times_ZB_over_Ld"
  Product/1 -> Add1/1
  [id_pu] -> Add1/2  "id_k_pu"
  [Rs_over_ZB_AXI] -> Product1/1  "Rs_over_ZB"
  [id_pu] -> Product1/2  "id_k_pu"
  [iq_pu] -> Product3/1  "iq_k_pu"
  [Lq_over_LB_AXI] -> Product3/2  "Lq_over_LB"
  [omega_m_pu] -> Product4/1  "omega_m_pu"
  [polepairs_AXI] -> Product4/2  "polepairs"
  [Ts_times_ZB_over_Lq_AXI] -> Product5/1  "Ts_times_ZB_over_Lq"
  [iq_pu] -> Product6/2  "iq_k_pu"
  [Rs_over_ZB_AXI] -> Product6/1  "Rs_over_ZB"
  Add2/1 -> Product5/2
  [omega_m_pu] -> Product9/1  "omega_m_pu"
  [iq_pu] -> Add3/2  "iq_k_pu"
  [id_pu] -> Product8/1  "id_k_pu"
  [Ld_over_LB_AXI] -> Product8/2  "Ld_over_LB"
  [polepairs_AXI] -> Product9/2  "polepairs"
  Product5/1 -> Add3/1
  [psi_pm_over_psiB_AXI] -> Product10/1
  [Ts_times_ZB_over_Lx_AXI] -> Product11/1  "Ts_times_ZB_over_Lx"
  [ix_pu] -> Product12/2  "ix_k_pu"
  [Rs_over_ZB_AXI] -> Product12/1  "Rs_over_ZB"
  Add4/1 -> Product11/2
  [ix_pu] -> Add5/2  "ix_k_pu"
  Product11/1 -> Add5/1
  [Rs_over_ZB_AXI] -> Product14/1  "Rs_over_ZB"
  Add6/1 -> Product13/2
  [iy_pu] -> Add7/2  "iy_k_pu"
  [iy_pu] -> Product14/2  "iy_k_pu"
  [Ts_times_ZB_over_Ly_AXI] -> Product13/1  "Ts_times_ZB_over_Ly"
  Product13/1 -> Add7/1
  Product2/1 -> Delay1/1
  Product1/1 -> Delay10/1
  Delay10/1 -> Add/2
  Delay1/1 -> Add/3
  [vd_pu] -> Delay18/1  "vd_pu"
  Delay18/1 -> Add/1
  [vq_pu] -> Delay19/1  "vq_pu"
  Product7/1 -> Delay21/1
  Product10/1 -> Delay22/1
  Delay22/1 -> Add2/4
  Delay21/1 -> Add2/3
  Delay20/1 -> Add2/2
  Delay19/1 -> Add2/1
  Product6/1 -> Delay20/1
  [vx_pu] -> Delay23/1  "vx_pu"
  Delay23/1 -> Add4/1
  Product12/1 -> Delay24/1
  Delay24/1 -> Add4/2
  [vy_pu] -> Delay41/1  "vy_pu"
  Product14/1 -> Delay42/1
  Delay42/1 -> Add6/2
  Delay41/1 -> Add6/1
  Product4/1 -> Delay45/1
  Product3/1 -> Delay46/1
  Delay46/1 -> Product2/2
  Delay45/1 -> Product2/1
  Product9/1 -> Delay47/1
  Delay47/1 -> Product10/2, Product7/1
  Product8/1 -> Delay48/1
  Delay48/1 -> Product7/2
  Detect Rise Positive1/1 -> Delay11/1, Switch31/2, Switch30/2, Switch29/2, Scope/3, Switch28/2  "delay_comp done"
  trigger_prediction/1 -> Delay50/1
  Delay50/1 -> Detect Rise Positive1/1
  Detect Rise Positive/1 -> Switch21/2, Switch19/2, Switch18/2, Switch17/2, Switch16/2, Switch15/2, Switch14/2, Switch13/2, Switch12/2, Switch5/2, Switch3/2, Switch2/2, Switch1/2, Scope/4, Switch/2

== system external_state_machine/pu_omega_m ==
  in1 : Inport  OutDataTypeStr=fixdt(1,24,11)
  AXI_pu_conv_in : Inport  Port=2  OutDataTypeStr=fixdt(0,18,18)
  adc_valid_trigger : Inport  Port=3  OutDataTypeStr=boolean
  Delay{32,64,127..129} (5 alike) : Delay
  Delay31 : Delay  DelayLength=1
  Detect Rise Positive : simulink/Logic and Bit Operations/Detect Rise Positive  vinit=0  OutDataTypeStr=boolean
  Product23 : Product  OutDataTypeStr=fixdt(1,24,11)
  Switch31 : Switch  Criteria=u2 > Threshold
  out1 : Outport
  pu_conv_done : Outport  Port=2  OutDataTypeStr=boolean  LockScale=on
  out1_AXI : Outport  Port=3
  wires:
  adc_valid_trigger/1 -> Delay32/1
  in1/1 -> Delay64/1
  Delay129/1 -> pu_conv_done/1
  AXI_pu_conv_in/1 -> Product23/1
  Delay64/1 -> Switch31/1
  Delay128/1 -> out1_AXI/1
  Delay32/1 -> Detect Rise Positive/1
  Switch31/1 -> Product23/2, Delay31/1
  Delay31/1 -> Switch31/3
  Detect Rise Positive/1 -> Delay129/1, Switch31/2
  Product23/1 -> Delay127/1, Delay128/1
  Delay127/1 -> out1/1

== system external_state_machine/pu_omega_m1 ==
  in1 : Inport  OutDataTypeStr=fixdt(1,24,11)
  AXI_pu_conv_in : Inport  Port=2  OutDataTypeStr=fixdt(0,18,18)
  adc_valid_trigger : Inport  Port=3  OutDataTypeStr=boolean
  Delay{32,64,127..129} (5 alike) : Delay
  Delay31 : Delay  DelayLength=1
  Detect Rise Positive : simulink/Logic and Bit Operations/Detect Rise Positive  vinit=0  OutDataTypeStr=boolean
  Product23 : Product  OutDataTypeStr=fixdt(1,24,11)
  Switch31 : Switch  Criteria=u2 > Threshold
  out1 : Outport
  pu_conv_done : Outport  Port=2  OutDataTypeStr=boolean  LockScale=on
  out1_AXI : Outport  Port=3
  wires:
  adc_valid_trigger/1 -> Delay32/1
  in1/1 -> Delay64/1
  Delay129/1 -> pu_conv_done/1
  AXI_pu_conv_in/1 -> Product23/1
  Delay64/1 -> Switch31/1
  Delay128/1 -> out1_AXI/1
  Delay32/1 -> Detect Rise Positive/1
  Switch31/1 -> Product23/2, Delay31/1
  Delay31/1 -> Switch31/3
  Detect Rise Positive/1 -> Delay129/1, Switch31/2
  Product23/1 -> Delay127/1, Delay128/1
  Delay127/1 -> out1/1

== system external_state_machine/pu_voltages_vsd ==
  note: 0=AXI 1=PL
  v_DC_pu : Inport  OutDataTypeStr=fixdt_type_constants
  sin_angle : Inport  Port=2  OutDataTypeStr=fixdt_type_sin_cos
  cos_angle : Inport  Port=3  OutDataTypeStr=fixdt_type_sin_cos
  index : Inport  Port=4
  index_select_AXI : Inport  Port=5
  index_AXI : Inport  Port=6
  trigger_park_done : Inport  Port=7
  trigger_voltages : Inport  Port=8
  Delay{,1,4..7,9..11,17..21} (14 alike) : Delay
  Delay12 : Delay  InitialCondition=1
  Delay13 : Delay  InitialCondition=1
  Delay14 : Delay  DelayLength=1  InitialCondition=1
  Delay15 : Delay  InitialCondition=1
  Delay16 : Delay  DelayLength=1  InitialCondition=1
  Delay2 : Delay  DelayLength=1
  Delay3 : Delay  DelayLength=1
  Delay56 : Delay  DelayLength=1
  Delay8 : Delay  DelayLength=1  InitialCondition=1
  Detect Rise Positive : simulink/Logic and Bit Operations/Detect Rise Positive  vinit=0  OutDataTypeStr=boolean
  Detect Rise Positive1 : simulink/Logic and Bit Operations/Detect Rise Positive  vinit=0  OutDataTypeStr=boolean
  Scope : Scope  NumInputPorts=2
  Switch : Switch  Criteria=u2 > Threshold
  Switch1 : Switch  Criteria=u2 > Threshold  OutDataTypeStr=fixdt_type_sin_cos
  Switch2 : Switch  Criteria=u2 > Threshold  OutDataTypeStr=fixdt_type_sin_cos
  Switch27 : Switch  Criteria=u2 > Threshold  OutDataTypeStr=fixdt_type_constants
  Switch3 : Switch  Criteria=u2 > Threshold  OutDataTypeStr=fixdt_type_polepairs
  Switch4 : Switch  Criteria=u2 > Threshold  OutDataTypeStr=fixdt_type_polepairs
  Switch5 : Switch  Criteria=u2 > Threshold  OutDataTypeStr=fixdt_type_polepairs
  finite_control_set : MATLAB Function  TreatAsAtomicUnit=on
  pu_vd : Outport
  pu_vq : Outport  Port=2
  pu_vx : Outport  Port=3
  pu_vy : Outport  Port=4
  pu_vd_AXI : Outport  Port=5
  pu_vq_AXI : Outport  Port=6
  pu_vx_AXI : Outport  Port=7
  pu_vy_AXI : Outport  Port=8
  voltages_done : Outport  Port=9
  wires:
  finite_control_set/1(pu_ud) -> Delay20/1, Delay7/1
  finite_control_set/2(pu_uq) -> Delay19/1, Delay6/1
  finite_control_set/3(pu_ux) -> Delay18/1, Delay5/1
  finite_control_set/4(pu_uy) -> Delay17/1, Delay4/1
  trigger_park_done/1 -> Delay/1
  Delay/1 -> Detect Rise Positive/1
  Delay56/1 -> Switch27/3
  v_DC_pu/1 -> Delay9/1
  Switch27/1 -> Delay56/1, finite_control_set/1(v_DC_pu)
  sin_angle/1 -> Delay10/1
  Delay2/1 -> Switch1/3
  Switch1/1 -> finite_control_set/2(sin_angle), Delay2/1
  cos_angle/1 -> Delay11/1
  Delay3/1 -> Switch2/3
  Switch2/1 -> finite_control_set/3(cos_angle), Delay3/1
  Delay4/1 -> pu_vy/1
  Delay5/1 -> pu_vx/1
  Delay6/1 -> pu_vq/1
  Delay7/1 -> pu_vd/1
  Switch3/1 -> Delay8/1, Switch/1
  index/1 -> Delay12/1
  Delay8/1 -> Switch3/3
  Delay9/1 -> Switch27/1
  Delay10/1 -> Switch1/1
  Delay11/1 -> Switch2/1
  Delay12/1 -> Switch3/1
  Delay14/1 -> Switch4/3
  index_AXI/1 -> Delay13/1
  Switch4/1 -> Switch/3, Delay14/1
  Delay13/1 -> Switch4/1
  Delay16/1 -> Switch5/3
  index_select_AXI/1 -> Delay15/1
  Switch5/1 -> Switch/2, Delay16/1
  Delay15/1 -> Switch5/1
  Delay17/1 -> pu_vy_AXI/1
  Delay19/1 -> pu_vq_AXI/1
  Delay20/1 -> pu_vd_AXI/1
  Delay18/1 -> pu_vx_AXI/1
  Detect Rise Positive1/1 -> Scope/2, Switch3/2, Switch4/2, Delay1/1  "trigger"
  Delay1/1 -> voltages_done/1
  Detect Rise Positive/1 -> Switch5/2, Switch2/2, Switch1/2, Switch27/2
  trigger_voltages/1 -> Delay21/1
  Delay21/1 -> Detect Rise Positive1/1
  Switch/1 -> Scope/1, finite_control_set/4(index)

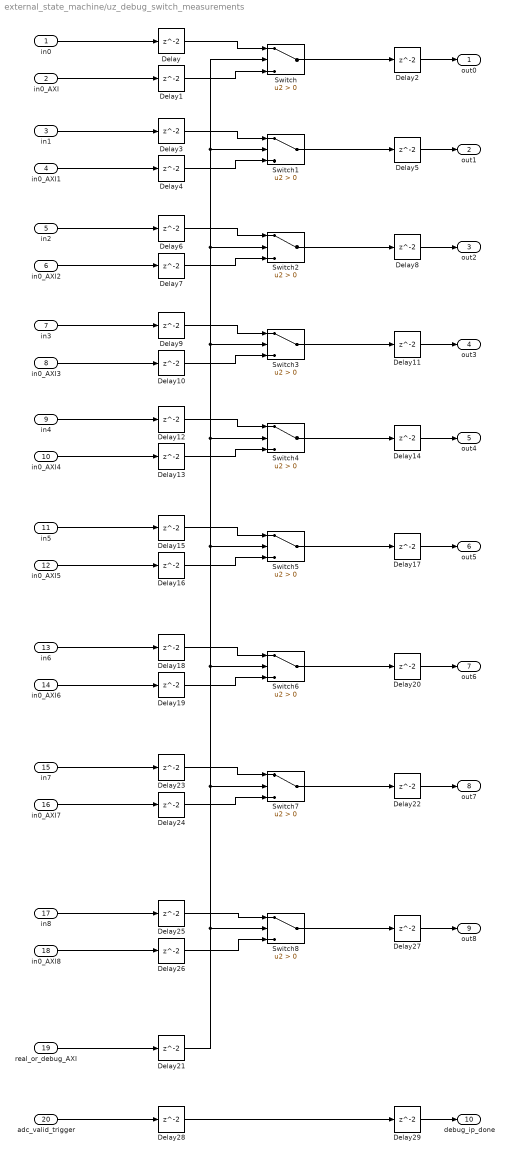
== system external_state_machine/uz_debug_switch_measurements ==
  in0 : Inport
  in0_AXI : Inport  Port=2
  in1 : Inport  Port=3
  in0_AXI1 : Inport  Port=4
  in2 : Inport  Port=5
  in0_AXI2 : Inport  Port=6
  in3 : Inport  Port=7
  in0_AXI3 : Inport  Port=8
  in4 : Inport  Port=9
  in0_AXI4 : Inport  Port=10
  in5 : Inport  Port=11
  in0_AXI5 : Inport  Port=12
  in6 : Inport  Port=13
  in0_AXI6 : Inport  Port=14
  in7 : Inport  Port=15
  in0_AXI7 : Inport  Port=16
  in8 : Inport  Port=17
  in0_AXI8 : Inport  Port=18
  real_or_debug_AXI : Inport  Port=19
  adc_valid_trigger : Inport  Port=20
  Delay{,1..29} (30 alike) : Delay
  Switch{,1..8} (9 alike) : Switch  Criteria=u2 > Threshold
  out0 : Outport  VectorParamsAs1DForOutWhenUnconnected=off
  out1 : Outport  Port=2  VectorParamsAs1DForOutWhenUnconnected=off
  out2 : Outport  Port=3  VectorParamsAs1DForOutWhenUnconnected=off
  out3 : Outport  Port=4  VectorParamsAs1DForOutWhenUnconnected=off
  out4 : Outport  Port=5  VectorParamsAs1DForOutWhenUnconnected=off
  out5 : Outport  Port=6  VectorParamsAs1DForOutWhenUnconnected=off
  out6 : Outport  Port=7  VectorParamsAs1DForOutWhenUnconnected=off
  out7 : Outport  Port=8  VectorParamsAs1DForOutWhenUnconnected=off
  out8 : Outport  Port=9  VectorParamsAs1DForOutWhenUnconnected=off
  debug_ip_done : Outport  Port=10  VectorParamsAs1DForOutWhenUnconnected=off
  wires:
  in0/1 -> Delay/1
  in0_AXI/1 -> Delay1/1
  Delay/1 -> Switch/1
  Delay1/1 -> Switch/3
  Switch/1 -> Delay2/1
  Delay2/1 -> out0/1
  in0_AXI1/1 -> Delay4/1
  Delay5/1 -> out1/1
  in1/1 -> Delay3/1
  Delay4/1 -> Switch1/3
  Delay3/1 -> Switch1/1
  Switch1/1 -> Delay5/1
  in0_AXI2/1 -> Delay7/1
  Delay8/1 -> out2/1
  in2/1 -> Delay6/1
  Delay7/1 -> Switch2/3
  Delay6/1 -> Switch2/1
  Switch2/1 -> Delay8/1
  in0_AXI3/1 -> Delay10/1
  Delay11/1 -> out3/1
  in3/1 -> Delay9/1
  Delay10/1 -> Switch3/3
  Delay9/1 -> Switch3/1
  Switch3/1 -> Delay11/1
  in0_AXI4/1 -> Delay13/1
  Delay14/1 -> out4/1
  in4/1 -> Delay12/1
  Delay13/1 -> Switch4/3
  Delay12/1 -> Switch4/1
  Switch4/1 -> Delay14/1
  in0_AXI5/1 -> Delay16/1
  Delay17/1 -> out5/1
  in5/1 -> Delay15/1
  Delay16/1 -> Switch5/3
  Delay15/1 -> Switch5/1
  Switch5/1 -> Delay17/1
  in0_AXI6/1 -> Delay19/1
  Delay20/1 -> out6/1
  in6/1 -> Delay18/1
  Delay19/1 -> Switch6/3
  Delay18/1 -> Switch6/1
  Switch6/1 -> Delay20/1
  real_or_debug_AXI/1 -> Delay21/1
  Delay22/1 -> out7/1
  Delay23/1 -> Switch7/1
  Delay24/1 -> Switch7/3
  Switch7/1 -> Delay22/1
  in0_AXI7/1 -> Delay24/1
  in7/1 -> Delay23/1
  in0_AXI8/1 -> Delay26/1
  in8/1 -> Delay25/1
  Delay27/1 -> out8/1
  Switch8/1 -> Delay27/1
  Delay25/1 -> Switch8/1
  Delay26/1 -> Switch8/3
  Delay21/1 -> Switch/2, Switch1/2, Switch2/2, Switch3/2, Switch4/2, Switch5/2, Switch6/2, Switch7/2, Switch8/2
  Delay28/1 -> Delay29/1
  Delay29/1 -> debug_ip_done/1
  adc_valid_trigger/1 -> Delay28/1
